simulink model "main_sl"  (R2023b)
settings: Solver=VariableStepAuto  StartTime=0.0  StopTime=10.0  RelTol=1e-3
settings Model: Creator=tard  LastModifiedBy=tard

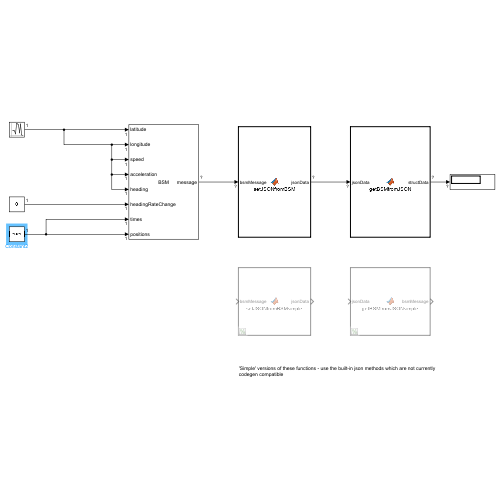
[thumbnail: Simulink's stored preview of the top-level diagram]
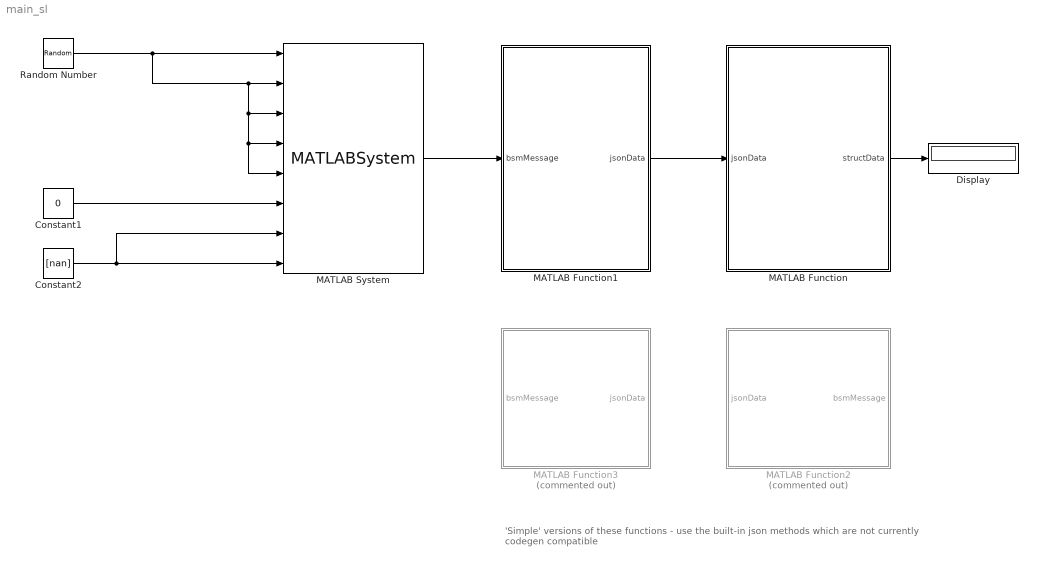
== system main_sl ==
  note: 'Simple' versions of these functions - use the built-in json methods which are not currently codegen compatible
  Constant1 : Constant  Value=0
  Constant2 : Constant  Value=[nan]
  Display : Display
  MATLAB Function : MATLAB Function  TreatAsAtomicUnit=on
  MATLAB Function1 : MATLAB Function  TreatAsAtomicUnit=on
  MATLAB Function2 : MATLAB Function  Commented=on  TreatAsAtomicUnit=on
  MATLAB Function3 : MATLAB Function  Commented=on  TreatAsAtomicUnit=on
  MATLAB System : MATLABSystem  System=BSM  requiredKeys={ 'current_utc_time', 'latitude', 'longitude', 'speed', 'acceleration', 'heading', 'heading_rate_change', 'error_flag' }  Defaults="struct( 'elevation', 0.0, 'position_accuracy', 1.5, 'steering_angle', 0.0, 'transmission_state', 'Drive', 'braking_status', false, 'turn_signal_status', 'Off', 'length', 4.2, 'width', 1.8, 'path_history', struct( 'rel_time', [  ], 'lateral_deviation', [  ], 'longitudinal_deviation', [  ] ), 'path_intentions', struct( 'rel_time', [  ], 'lateral_deviation', [  ], 'longitudinal_deviation', [  ] ) )"  SimulateUsing=Code generation
      mask Type: BSM
      mask Display:
      | disp('BSM');
      | port_label('input',1,'latitude');
      | port_label('input',2,'longitude');
      | port_label('input',3,'speed');
      | port_label('input',4,'acceleration');
      | port_label('input',5,'heading');
      | port_label('input',6,'headingRateChange');
      | port_label('input',7,'times');
      | port_label('input',8,'positions');
      | port_label('output',1,'message');
  Random Number : RandomNumber  SampleTime=0.1
  wires:
  Random Number/1 -> MATLAB System/5, MATLAB System/4, MATLAB System/3, MATLAB System/2, MATLAB System/1
  Constant2/1 -> MATLAB System/8, MATLAB System/7
  Constant1/1 -> MATLAB System/6
  MATLAB System/1 -> MATLAB Function1/1(bsmMessage)
  MATLAB Function1/1(jsonData) -> MATLAB Function/1(jsonData)
  MATLAB Function/1(structData) -> Display/1

== matlab function main_sl/MATLAB Function ==
  data: jsonData input; structData output
%%%%%%%%%%%%%%%%%%%%%%%%%%%%%%%%%%%%%%%
%%% Tyler Ard                       %%%
%%% Vehicle Mobility Systems Group  %%%
%%% tard(at)anl(dot)gov             %%%
%%%%%%%%%%%%%%%%%%%%%%%%%%%%%%%%%%%%%%%


function structData = getBSMfromJSON(jsonData)
    %#codegen
    % Parses JSON string manually into a structured format for Simulink & MATLAB CodeGen.

    coder.varsize('jsonData', [1, 2000]);

    % Ensure input is a string
    assert(ischar(jsonData) || isstring(jsonData), 'Input must be a valid JSON string.');

    % Initialize default struct with expected fields
    max_vector_len = 100;

    structData = struct( ...
        'current_utc_time', 0.0, ...
        'latitude', 0.0, ...
        'longitude', 0.0, ...
        'speed', 0.0, ...
        'acceleration', 0.0, ...
        'heading', 0.0, ...
        'heading_rate_change', 0.0, ...
        'error_flag', "OK", ...
        'path_history', struct('rel_time', nan(max_vector_len,1), 'lateral_deviation', nan(max_vector_len,1), 'longitudinal_deviation', nan(max_vector_len,1)), ...
        'path_intentions', struct('rel_time', nan(max_vector_len,1), 'lateral_deviation', nan(max_vector_len,1), 'longitudinal_deviation', nan(max_vector_len,1)) ...
    );

    % Extract numeric values using manual parsing (C/C++ compatible)
    structData.current_utc_time = extractNumeric(jsonData, '"current_utc_time":');
    structData.latitude = extractNumeric(jsonData, '"latitude":');
    structData.longitude = extractNumeric(jsonData, '"longitude":');
    structData.speed = extractNumeric(jsonData, '"speed":');
    structData.acceleration = extractNumeric(jsonData, '"acceleration":');
    structData.heading = extractNumeric(jsonData, '"heading":');
    structData.heading_rate_change = extractNumeric(jsonData, '"heading_rate_change":');

    % Extract error flag as a character string
    structData.error_flag = extractString(jsonData, '"error_flag":"');

    % Extract path history arrays
    path_history = extractNestedJson(jsonData, '"path_history":');
    
    structData.path_history.rel_time = extractArray(path_history, '"rel_time":[', max_vector_len);
    structData.path_history.lateral_deviation = extractArray(path_history, '"lateral_deviation":[', max_vector_len);
    structData.path_history.longitudinal_deviation = extractArray(path_history, '"longitudinal_deviation":[', max_vector_len);

    % Extract path intentions arrays
    path_intentions = extractNestedJson(jsonData, '"path_intentions":');

    structData.path_intentions.rel_time = extractArray(path_intentions, '"rel_time":[', max_vector_len);
    structData.path_intentions.lateral_deviation = extractArray(path_intentions, '"lateral_deviation":[', max_vector_len);
    structData.path_intentions.longitudinal_deviation = extractArray(path_intentions, '"longitudinal_deviation":[', max_vector_len);
end

function value = extractNumeric(jsonStr, fieldName)
    %#codegen
    % Extracts a numeric value from a JSON string.
    
    startIdx = strfind(jsonStr, fieldName);
    if isempty(startIdx)
        value = 0.0;
        return;
    end
    
    startIdx = startIdx + length(fieldName);
    endIdx = strfind(jsonStr(startIdx:end), ',') + startIdx - 2;
    if isempty(endIdx)
        endIdx = strfind(jsonStr(startIdx:end), '}') + startIdx - 2;
    end
    
    value = str2double(jsonStr(startIdx:endIdx));
end

function value = extractString(jsonStr, fieldName)
    %#codegen
    % Extracts a string value from a JSON string.
    
    startIdx = strfind(jsonStr, fieldName);
    if isempty(startIdx)
        value = ""; % Default
        return;
    end
    
    startIdx = startIdx + length(fieldName);
    endIdx = strfind(jsonStr(startIdx:end), '"') + startIdx - 2;
    
    value = jsonStr(startIdx:endIdx);
end

function json = extractNestedJson(jsonStr, fieldName)
    %#codegen
    % Extracts a sub JSON field from a JSON string.
    
    startIdx = strfind(jsonStr, fieldName);
    if isempty(startIdx)
        value = "{}";
        return;
    end
    
    startIdx = startIdx + length(fieldName);
    endIdx = strfind(jsonStr(startIdx:end), '}') + startIdx - 1;
    if isempty(endIdx)
        endIdx = strfind(jsonStr(startIdx:end), ',') + startIdx - 2;
    end
    
    json = jsonStr(startIdx:endIdx);
end

function values = extractArray(jsonStr, fieldName, max_vector_len)
    %#codegen
    % Extracts a numeric array from a JSON string while ensuring fixed-size compatibility.

    startIdx = strfind(jsonStr, fieldName);
    if isempty(startIdx)
        values = nan(max_vector_len, 1);
        return;
    end

    startIdx = startIdx + length(fieldName);
    endIdx = strfind(jsonStr(startIdx:end), ']') + startIdx - 2;

    % Convert extracted substring into numeric array
    numStr = jsonStr(startIdx:endIdx);
    strValues = str2double(split(numStr, ','));

    % Ensure fixed-size compatibility using direct indexing
    values = nan(max_vector_len, 1); % Preallocate 
    numEntries = min(length(strValues), max_vector_len);

    values(1:numEntries) = strValues(1:numEntries);
end

== matlab function main_sl/MATLAB Function2 ==
  data: jsonData input; bsmMessage output
%%%%%%%%%%%%%%%%%%%%%%%%%%%%%%%%%%%%%%%
%%% Tyler Ard                       %%%
%%% Vehicle Mobility Systems Group  %%%
%%% tard(at)anl(dot)gov             %%%
%%%%%%%%%%%%%%%%%%%%%%%%%%%%%%%%%%%%%%%

function bsmMessage = getBSMfromJSONsimple(jsonData)
    % Converts a JSON message to BSM message struct.
    %
    % Outputs:
    %   jsonData - JSON formatted string.
    %
    % Inputs:
    %   bsmMessage - Struct containing the BSM data with fixed fields.
    
    bsmMessage = jsondecode(jsonData);
end

== matlab function main_sl/MATLAB Function3 ==
  data: bsmMessage input; jsonData output
%%%%%%%%%%%%%%%%%%%%%%%%%%%%%%%%%%%%%%%
%%% Tyler Ard                       %%%
%%% Vehicle Mobility Systems Group  %%%
%%% tard(at)anl(dot)gov             %%%
%%%%%%%%%%%%%%%%%%%%%%%%%%%%%%%%%%%%%%%

function jsonData = setJSONfromBSMsimple(bsmMessage)
    % Converts a BSM message struct to JSON format.
    %
    % Inputs:
    %   bsmMessage - Struct containing the BSM data with fixed fields.
    %
    % Outputs:
    %   jsonData - JSON formatted string.

    % Validate input type
    if ~isstruct(bsmMessage)
        error('Input must be a struct containing BSM data.');
    end
    
    % Ensure path history and path intentions are correctly formatted
    jsonData = jsonencode(bsmMessage);
end

== matlab function main_sl/MATLAB Function1 ==
  data: bsmMessage input; jsonData output
%%%%%%%%%%%%%%%%%%%%%%%%%%%%%%%%%%%%%%%
%%% Tyler Ard                       %%%
%%% Vehicle Mobility Systems Group  %%%
%%% tard(at)anl(dot)gov             %%%
%%%%%%%%%%%%%%%%%%%%%%%%%%%%%%%%%%%%%%%

function jsonData = setJSONfromBSM(bsmMessage)
    %#codegen
    % Converts a BSM message struct to JSON format for Simulink & C Code Generation.
    %
    % Inputs:
    %   bsmMessage - Struct containing the BSM data with fixed fields.
    %
    % Outputs:
    %   jsonData - JSON formatted string.

    coder.varsize('jsonData', [1, 2000]); % Specifies y as variable-size with max dimensions [1, n]

    coder.varsize('pathIntentionsJSON', [1, 2000]); % Specifies y as variable-size with max dimensions [1, n]
    coder.varsize('pathHistoryJSON', [1, 2000]); % Specifies y as variable-size with max dimensions [1, n]

    jsonData = blanks(2000);
    pathIntentionsJSON = blanks(2000);
    PathHistoryJSON = blanks(2000);

    % Validate input type
    if ~isstruct(bsmMessage)
        error('Input must be a struct containing BSM data.');
    end
    
    % Ensure path history and path intentions are correctly formatted
    if ~isfield(bsmMessage, 'path_history')
        bsmMessage.path_history = struct('rel_time', [], 'lateral_deviation', [], 'longitudinal_deviation', []);
    end
    if ~isfield(bsmMessage, 'path_intentions')
        bsmMessage.path_intentions = struct('rel_time', [], 'lateral_deviation', [], 'longitudinal_deviation', []);
    end
    
    %%% NUM2STR FUNCTION IS NOT CODEGEN COMPATIBLE
    % % Convert path history and path intentions to JSON-compatible format
    % pathHistoryJSON = sprintf('{\"rel_time\":[%s],\"lateral_deviation\":[%s],\"longitudinal_deviation\":[%s]}', ...
    %     num2str(bsmMessage.path_history.rel_time, '%.6f,'), ...
    %     num2str(bsmMessage.path_history.lateral_deviation, '%.6f,'), ...
    %     num2str(bsmMessage.path_history.longitudinal_deviation, '%.6f,'));
    % 
    % pathIntentionsJSON = sprintf('{\"rel_time\":[%s],\"lateral_deviation\":[%s],\"longitudinal_deviation\":[%s]}', ...
    %     num2str(bsmMessage.path_intentions.rel_time, '%.6f,'), ...
    %     num2str(bsmMessage.path_intentions.lateral_deviation, '%.6f,'), ...
    %     num2str(bsmMessage.path_intentions.longitudinal_deviation, '%.6f,'));
    % 
    % % Manually construct the full JSON string
    % jsonData = sprintf('{\"current_utc_time\":%.6f, \"latitude\":%.6f, \"longitude\":%.6f, \"speed\":%.2f, \"acceleration\":%.2f, \"heading\":%.6f, \"heading_rate_change\":%.6f, \"error_flag\":\"%s\", \"path_history\":%s, \"path_intentions\":%s}', ...
    %     bsmMessage.current_utc_time, bsmMessage.latitude, bsmMessage.longitude, ...
    %     bsmMessage.speed, bsmMessage.acceleration, bsmMessage.heading, ...
    %     bsmMessage.heading_rate_change, bsmMessage.error_flag, ...
    %     pathHistoryJSON, pathIntentionsJSON);

    % Convert path history and path intentions to JSON-compatible format
    pathHistoryJSONtmp = sprintf('{\"rel_time\":[%s],\"lateral_deviation\":[%s],\"longitudinal_deviation\":[%s]}', ...
        formatArrayForJSON(bsmMessage.path_history.rel_time, '%.6f'), ...
        formatArrayForJSON(bsmMessage.path_history.lateral_deviation, '%.6f'), ...
        formatArrayForJSON(bsmMessage.path_history.longitudinal_deviation, '%.6f'));

    pathIntentionsJSONtmp = sprintf('{\"rel_time\":[%s],\"lateral_deviation\":[%s],\"longitudinal_deviation\":[%s]}', ...
        formatArrayForJSON(bsmMessage.path_intentions.rel_time, '%.6f'), ...
        formatArrayForJSON(bsmMessage.path_intentions.lateral_deviation, '%.6f'), ...
        formatArrayForJSON(bsmMessage.path_intentions.longitudinal_deviation, '%.6f'));

    pathHistoryJSON(1:length(pathHistoryJSONtmp)) = pathHistoryJSONtmp(:);
    pathIntentionsJSON(1:length(pathIntentionsJSONtmp)) = pathIntentionsJSONtmp(:);

    % Manually construct the full JSON string
    jsonDatatmp = sprintf('{\"current_utc_time\":%.6f, \"latitude\":%.6f, \"longitude\":%.6f, \"speed\":%.2f, \"acceleration\":%.2f, \"heading\":%.6f, \"heading_rate_change\":%.6f, \"error_flag\":\"%s\", \"path_history\":%s, \"path_intentions\":%s}', ...
        bsmMessage.current_utc_time, bsmMessage.latitude, bsmMessage.longitude, ...
        bsmMessage.speed, bsmMessage.acceleration, bsmMessage.heading, ...
        bsmMessage.heading_rate_change, bsmMessage.error_flag, ...
        pathHistoryJSON, pathIntentionsJSON);

    jsonData(1:length(jsonDatatmp)) = jsonDatatmp(:);
end

% Helper function for formatting arrays without num2str
function formattedStr = formatArrayForJSON(array, formatSpec)
    %#codegen
    % Converts a numeric array into a JSON-compatible formatted string.
    
    formattedStr = '';
    for i = 1:length(array)
        formattedStr = [formattedStr, sprintf(formatSpec, array(i))];
        if i < length(array)
            formattedStr = [formattedStr, ',']; % Add comma separator
        end
    end
end
